simulink model "mechdyn"  (R2015a)
settings: Solver=ode45  StartTime=0.0  StopTime=10.0  RelTol=1e-3
undefined symbols (not defined in the file): bu_tot, kx_l, m_tot
settings Model: Creator=Heath  LastModifiedBy=Hofmann
settings DataIOCC: SignalLoggingSaveFormat=ModelDataLogs
settings OptimizationCC: ExpressionDepthLimit=2147483647
settings DebuggingCC: UnderspecifiedInitializationDetection=Classic  MergeDetectMultiDrivingBlocksExec=none  SolverPrmCheckMsg=warning  BusObjectLabelMismatch=error  StateNameClashWarn=warning  StrictBusMsg=Warning
settings GRTTargetCC: CombineOutputUpdateFcns=off  GRTInterface=on

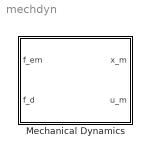
== system mechdyn ==
  Mechanical Dynamics : Subsystem

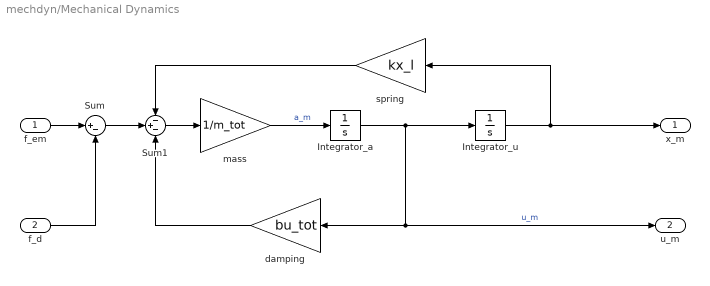
== system mechdyn/Mechanical Dynamics ==
  f_em : Inport
  f_d : Inport  Port=2
  Integrator_a : Integrator
  Integrator_u : Integrator
  Sum : Sum  Inputs=|+-
  Sum1 : Sum  Inputs=-+-
  damping : Gain  Gain=bu_tot
  mass : Gain  Gain=1/m_tot
  spring : Gain  Gain=kx_l
  x_m : Outport
  u_m : Outport  Port=2
  wires:
  f_em/1 -> Sum/1
  f_d/1 -> Sum/2
  mass/1 -> Integrator_a/1  "a_m"
  Integrator_a/1 -> Integrator_u/1, u_m/1, damping/1  "u_m"
  Integrator_u/1 -> x_m/1, spring/1
  Sum/1 -> Sum1/2
  Sum1/1 -> mass/1
  damping/1 -> Sum1/3
  spring/1 -> Sum1/1
